simulink model "0_modelo_sensor"  (R2021a)
settings: Solver=VariableStepAuto  StartTime=0.0  StopTime=10.0  RelTol=1e-3
libraries: simulink x2
settings Model: Creator=temis  LastModifiedBy=temis

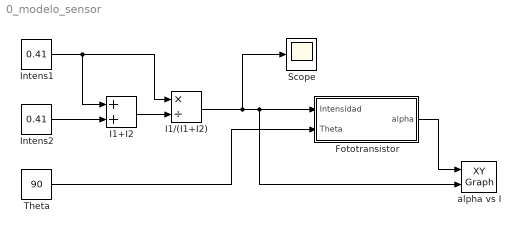
== system 0_modelo_sensor ==
  Fototransistor : Subsystem
  I1+I2 : Sum
  I1/(I1+I2) : Product  Inputs=*/
  Intens1 : Constant  Value=0.41
  Intens2 : Constant  Value=0.41
  Scope : Scope
  Theta : Constant  Value=90
  alpha vs I : simulink/Sinks/XY Graph  xmin=-1  xmax=1  ymin=-1  ymax=1  st=-1
  wires:
  Fototransistor/1(alpha) -> alpha vs I/1
  I1/(I1+I2)/1 -> Scope/1, alpha vs I/2, Fototransistor/1(Intensidad)
  Theta/1 -> Fototransistor/2(Theta)
  Intens2/1 -> I1+I2/2
  I1+I2/1 -> I1/(I1+I2)/2
  Intens1/1 -> I1/(I1+I2)/1, I1+I2/1

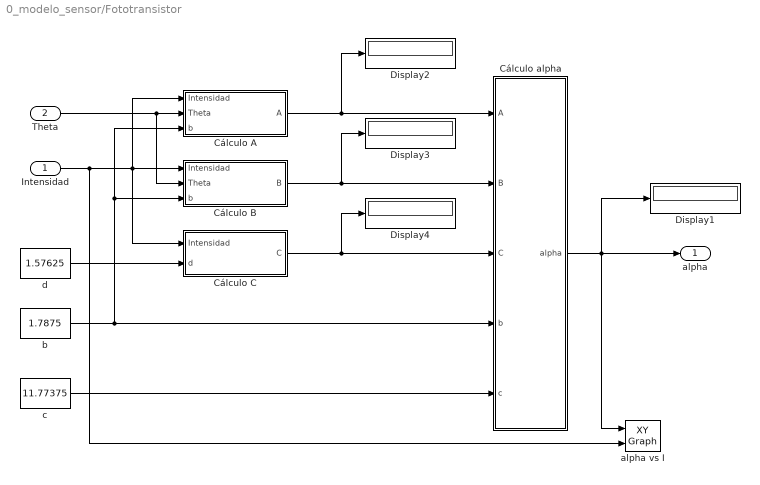
== system 0_modelo_sensor/Fototransistor ==
  Intensidad : Inport
  Theta : Inport  Port=2
  Cálculo A : Subsystem
  Cálculo B : Subsystem
  Cálculo C : Subsystem
  Cálculo alpha : MATLAB Function  TreatAsAtomicUnit=on
  Display{1..4} (4 alike) : Display
  alpha vs I : simulink/Sinks/XY Graph  xmin=-1  xmax=1  ymin=-1  ymax=1  st=-1
  b : Constant  Value=1.7875
  c : Constant  Value=11.77375
  d : Constant  Value=1.57625
  alpha : Outport
  wires:
  Cálculo C/1(C) -> Display4/1, Cálculo alpha/3(C)
  Cálculo alpha/1(alpha) -> Display1/1, alpha/1, alpha vs I/1
  Intensidad/1 -> Cálculo B/1(Intensidad), Cálculo A/1(Intensidad), Cálculo C/1(Intensidad), alpha vs I/2
  Theta/1 -> Cálculo B/2(Theta), Cálculo A/2(Theta)
  Cálculo B/1(B) -> Display3/1, Cálculo alpha/2(B)
  Cálculo A/1(A) -> Display2/1, Cálculo alpha/1(A)
  b/1 -> Cálculo alpha/4(b), Cálculo B/3(b), Cálculo A/3(b)
  c/1 -> Cálculo alpha/5(c)
  d/1 -> Cálculo C/2(d)

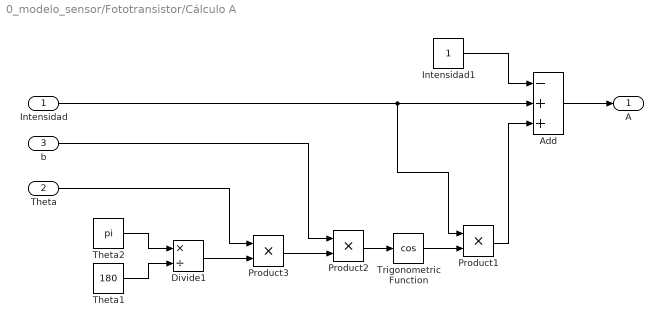
== system 0_modelo_sensor/Fototransistor/Cálculo A ==
  Intensidad : Inport
  Theta : Inport  Port=2
  b : Inport  Port=3
  Add : Sum  Inputs=-++
  Divide1 : Product  Inputs=*/
  Intensidad1 : Constant
  Product1 : Product
  Product2 : Product
  Product3 : Product
  Theta1 : Constant  Value=180
  Theta2 : Constant  Value=pi
  Trigonometric Function : Trigonometry  Operator=cos
  A : Outport
  wires:
  Divide1/1 -> Product3/2
  Product3/1 -> Product2/2
  Theta2/1 -> Divide1/1
  Intensidad1/1 -> Add/1
  Product1/1 -> Add/3
  Theta1/1 -> Divide1/2
  Trigonometric Function/1 -> Product1/2
  Product2/1 -> Trigonometric Function/1
  Intensidad/1 -> Product1/1, Add/2
  Theta/1 -> Product3/1
  Add/1 -> A/1
  b/1 -> Product2/1

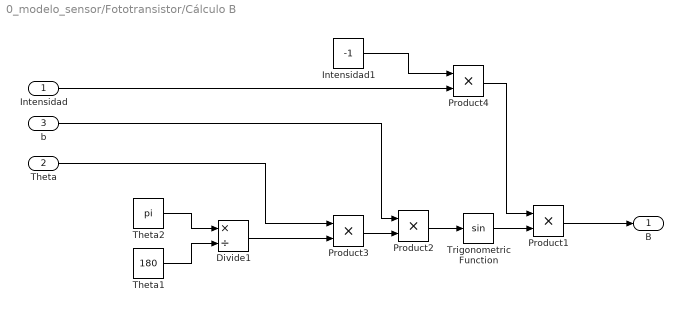
== system 0_modelo_sensor/Fototransistor/Cálculo B ==
  Intensidad : Inport
  Theta : Inport  Port=2
  b : Inport  Port=3
  Divide1 : Product  Inputs=*/
  Intensidad1 : Constant  Value=-1
  Product{1..4} (4 alike) : Product
  Theta1 : Constant  Value=180
  Theta2 : Constant  Value=pi
  Trigonometric Function : Trigonometry
  B : Outport
  wires:
  Divide1/1 -> Product3/2
  Product3/1 -> Product2/2
  Theta2/1 -> Divide1/1
  Product1/1 -> B/1
  Theta1/1 -> Divide1/2
  Trigonometric Function/1 -> Product1/2
  Product2/1 -> Trigonometric Function/1
  Intensidad/1 -> Product4/2
  Theta/1 -> Product3/1
  Intensidad1/1 -> Product4/1
  Product4/1 -> Product1/1
  b/1 -> Product2/1

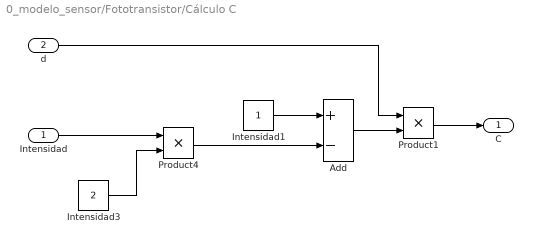
== system 0_modelo_sensor/Fototransistor/Cálculo C ==
  Intensidad : Inport
  d : Inport  Port=2
  Add : Sum  Inputs=+-
  Intensidad1 : Constant
  Intensidad3 : Constant  Value=2
  Product1 : Product
  Product4 : Product
  C : Outport
  wires:
  Intensidad1/1 -> Add/1
  Intensidad/1 -> Product4/1
  Intensidad3/1 -> Product4/2
  Product4/1 -> Add/2
  Add/1 -> Product1/2
  Product1/1 -> C/1
  d/1 -> Product1/1

== matlab function 0_modelo_sensor/Fototransistor/Cálculo alpha ==
  data: A input; alpha output; B input; C input; b input; c input
function alpha = fcn(A, B, C, b, c)

    if ((A+C ~= 0) && (-B*sqrt(A^2+B^2-C^2)+A^2+A*C+B^2 ~= 0))
        
        alpha = 2*atan((B-sqrt(A^2+B^2-C^2))/(A+C));

    elseif ((A+C ~= 0) && (B*sqrt(A^2+B^2-C^2)+A^2+A*C+B^2 ~= 0))

        alpha = 2*atan((B+sqrt(A^2+B^2-C^2))/(A+C));

    elseif ((B ~= 0) && (A^2+B^2~=0) && (C == -A))

        alpha = -2*atan(A/B);

    elseif (A == -C)

        alpha = pi;

    else

        alpha = 1000;

    end

    alpha = (alpha -c*pi/180)/b;

    alpha = alpha*180/pi;

end
